simulink model "EX4zadanie3"  (R2023b)
settings: Solver=FixedStepDiscrete  StartTime=0.0  StopTime=0.0  RelTol=1e-3
libraries: CPOiS_SourcesSinks x6, CPOiS_LinearTransforms x4, CPOiS_DataManipulation_DataTypeConversion x4
settings Model: Creator=kkarkosz  LastModifiedBy=alyskawa

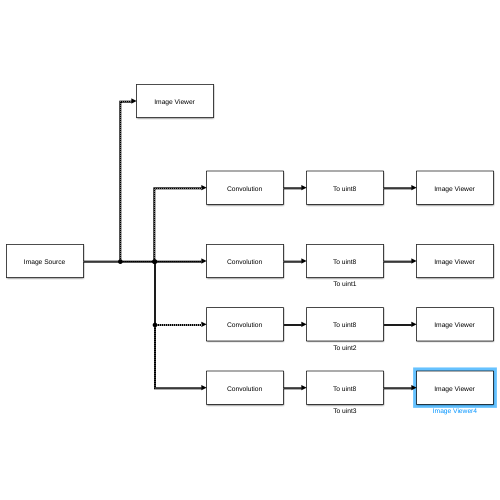
[thumbnail: Simulink's stored preview of the top-level diagram]
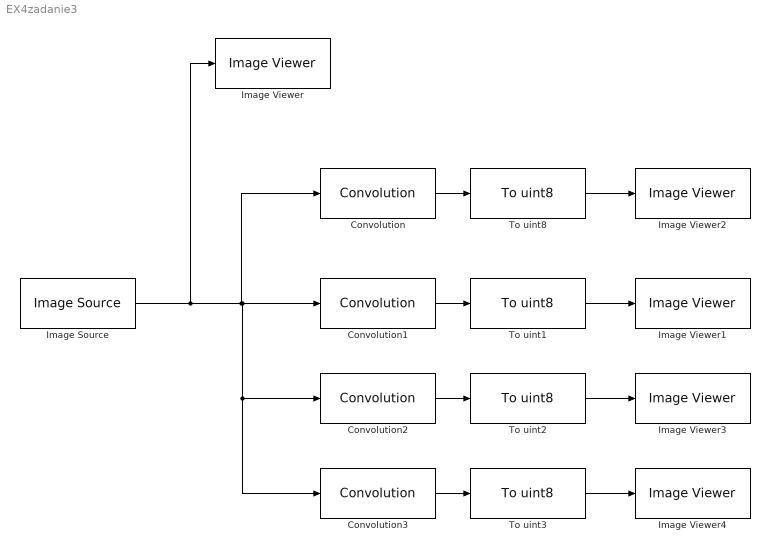
== system EX4zadanie3 ==
  Convolution : CPOiS_LinearTransforms/Convolution  ConvolutionMatrix=[1,0,-1;1,0,-1;1,0,-1]
      settings: SourceProductName=CPOiS - Digital image and signal processing
  Convolution1 : CPOiS_LinearTransforms/Convolution  ConvolutionMatrix=[1,1,1;0,0,0;-1,-1,-1]
      settings: SourceProductName=CPOiS - Digital image and signal processing
  Convolution2 : CPOiS_LinearTransforms/Convolution  ConvolutionMatrix=1/(sum(sum([1;4;5;0;-5;-4;-1] * [1;4;5;0;-5;-4;-1]'))) * [1;4;5;0;-5;-4;-1]* [1;4;5;0;-5;-4;-1]'
      settings: SourceProductName=CPOiS - Digital image and signal processing
  Convolution3 : CPOiS_LinearTransforms/Convolution  ConvolutionMatrix=[0,1,0;1,-4,1;0,1,0]
      settings: SourceProductName=CPOiS - Digital image and signal processing
  Image Source : CPOiS_SourcesSinks/Image Source  FileSelection=gull.png
      settings: SourceProductName=CPOiS - Digital image and signal processing
  Image Viewer{,1..4} (5 alike) : CPOiS_SourcesSinks/Image Viewer
      settings: SourceProductName=CPOiS - Digital image and signal processing
  To uint{1..3,8} (4 alike) : CPOiS_DataManipulation_DataTypeConversion/To uint8
      settings: SourceProductName=CPOiS - Digital image and signal processing
  wires:
  Convolution/1 -> To uint8/1
  To uint8/1 -> Image Viewer2/1
  Convolution1/1 -> To uint1/1
  To uint1/1 -> Image Viewer1/1
  To uint2/1 -> Image Viewer3/1
  Convolution2/1 -> To uint2/1
  Convolution3/1 -> To uint3/1
  To uint3/1 -> Image Viewer4/1
  Image Source/1 -> Image Viewer/1, Convolution3/1, Convolution2/1, Convolution1/1, Convolution/1
